simulink model "e2"  (R2014b)
settings: Solver=ode45  StartTime=0.0  StopTime=10.0  RelTol=1e-3
settings Model: Creator=Administrator  LastModifiedBy=Administrator

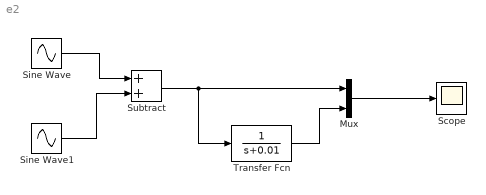
== system e2 ==
  Mux : Mux  Inputs=2
  Scope : Scope
  Sine Wave : Sin  SampleTime=0
  Sine Wave1 : Sin  Frequency=20  SampleTime=0
  Subtract : Sum
  Transfer Fcn : TransferFcn  Numerator=1  Denominator=[1 0.01]
  wires:
  Sine Wave/1 -> Subtract/1
  Sine Wave1/1 -> Subtract/2
  Subtract/1 -> Transfer Fcn/1, Mux/1
  Transfer Fcn/1 -> Mux/2
  Mux/1 -> Scope/1
